simulink model "Task3"  (R2018b)
settings: Solver=VariableStepAuto  StartTime=0.0  StopTime=50  MaxStep=1e-3  RelTol=1e-3
settings Model: Creator=Федор  LastModifiedBy=Федор

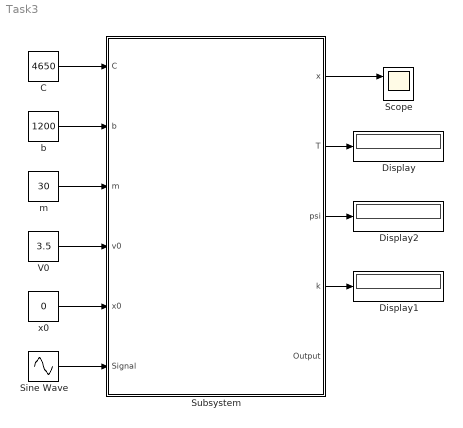
== system Task3 ==
  C : Constant  Value=4650
  Display : Display
  Display1 : Display
  Display2 : Display
  Scope : Scope  NumInputPorts=2
  Sine Wave : Sin  Amplitude=10000000  Frequency=4  SampleTime=0
  Subsystem : Subsystem
  "V0 " : Constant  Value=3.5
  b : Constant  Value=1200
  "m " : Constant  Value=30
  "x0 " : Constant  Value=0
  wires:
  C/1 -> Subsystem/1(C)
  b/1 -> Subsystem/2("b ")
  "m "/1 -> Subsystem/3(m)
  "V0 "/1 -> Subsystem/4(v0)
  "x0 "/1 -> Subsystem/5(x0)
  Sine Wave/1 -> Subsystem/6("Signal ")
  Subsystem/1(x) -> Scope/1
  Subsystem/2(T) -> Display/1
  Subsystem/3(psi) -> Display2/1
  Subsystem/4(k) -> Display1/1

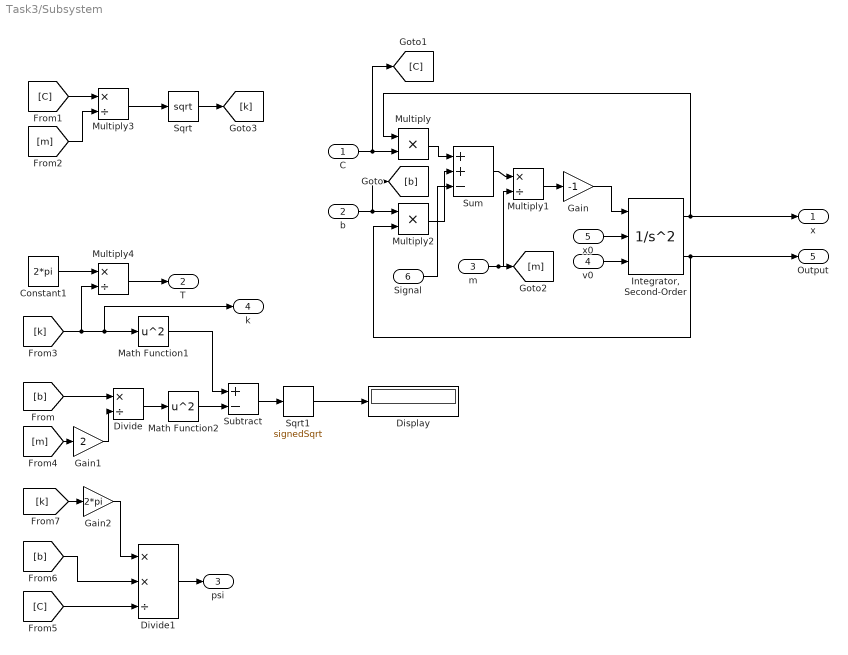
== system Task3/Subsystem ==
  C : Inport
  "b " : Inport  Port=2
  m : Inport  Port=3
  v0 : Inport  Port=4
  x0 : Inport  Port=5
  "Signal " : Inport  Port=6
  Constant1 : Constant  Value=2*pi
  Display : Display
  Divide : Product  Inputs=*/  OutDataTypeStr=double
  Divide1 : Product  Inputs=**/  OutDataTypeStr=double
  Gain : Gain  Gain=-1
  Gain1 : Gain  Gain=2
  Gain2 : Gain  Gain=2*pi
  "Integrator, Second-Order" : SecondOrderIntegrator  ICSourceX=external  ICSourceDXDT=external
  Math Function1 : Math  Operator=square  OutDataTypeStr=double  SaturateOnIntegerOverflow=on
  Math Function2 : Math  Operator=square  SaturateOnIntegerOverflow=on
  Multiply : Product
  Multiply1 : Product  Inputs=*/
  Multiply2 : Product
  Multiply3 : Product  Inputs=*/
  Multiply4 : Product  Inputs=*/
  Sqrt : Sqrt  SaturateOnIntegerOverflow=on
  Sqrt1 : Sqrt  Operator=signedSqrt  SaturateOnIntegerOverflow=on
  Subtract : Sum  Inputs=+-  OutDataTypeStr=double
  Sum : Sum  Inputs=++-
  x : Outport
  T : Outport  Port=2
  psi : Outport  Port=3
  k : Outport  Port=4
  Output : Outport  Port=5
  wires:
  Gain/1 -> "Integrator, Second-Order"/1
  "Integrator, Second-Order"/1 -> Multiply/1, x/1
  Multiply1/1 -> Gain/1
  m/1 -> Multiply1/2, [m]
  Multiply/1 -> Sum/1
  Multiply2/1 -> Sum/2
  Sum/1 -> Multiply1/1
  "Integrator, Second-Order"/2 -> Output/1, Multiply2/2
  v0/1 -> "Integrator, Second-Order"/3
  "Signal "/1 -> Sum/3
  "b "/1 -> [b], Multiply2/1
  C/1 -> [C], Multiply/2
  x0/1 -> "Integrator, Second-Order"/2
  [C] -> Multiply3/1
  [m] -> Multiply3/2
  Multiply3/1 -> Sqrt/1
  Sqrt/1 -> [k]
  Constant1/1 -> Multiply4/1
  Multiply4/1 -> T/1
  [k] -> k/1, Math Function1/1, Multiply4/2
  [m] -> Gain1/1
  [b] -> Divide/1
  Gain1/1 -> Divide/2
  Divide/1 -> Math Function2/1
  Math Function2/1 -> Subtract/2
  Subtract/1 -> Sqrt1/1
  Sqrt1/1 -> Display/1
  Gain2/1 -> Divide1/1
  [C] -> Divide1/3
  [b] -> Divide1/2
  Divide1/1 -> psi/1
  Math Function1/1 -> Subtract/1
  [k] -> Gain2/1
